simulink model "ata_xaui_2048pt_w32pnk"  (Simulink 6.2)
settings: Solver=ode45  StartTime=0.0  StopTime=20000  RelTol=1e-3
undefined symbols (not defined in the file): iBOB, pfb_coeff_gen_calc
libraries: xbsIndex_r3 x326, casper_library x37, xps_library x31, fft_library x1
(part 1 of 3)
settings Model: LastModifiedBy=siemion
settings DebuggingCC: SolverPrmCheckMsg=warning

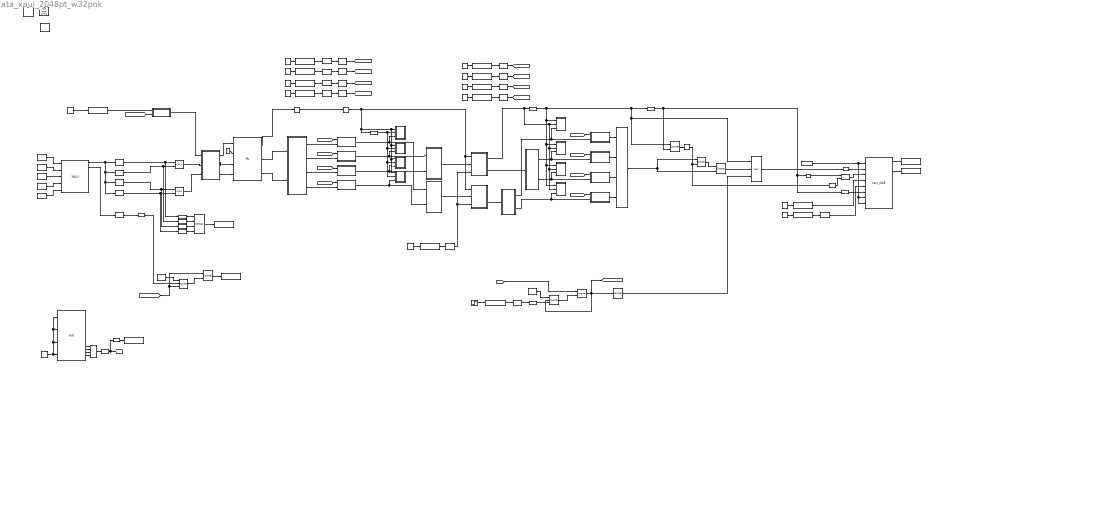
== system ata_xaui_2048pt_w32pnk ==
  note: left
  note: ATA Pulsar Machine
      | Author: Peter McMahon
      | Version: 1.0
      | February 2008
  note: n * LCM(taps*clksperFFT=2*2048=4096,
      | clksperacc=(acclen+1)*veclen=5*2048=10240)=20480
  note: XAUI Output:
      |
      | outofband[0]: 100PPS
      | outofband[1]: 1PPS
      |
      | data[0-7]: Pol 1 I
      | data[8-15]: Pol 1 Q
      | data[16-23]: Pol 2 I
      | data[24-31]: Pol 2 Q
      | data[31-63]: unused
  note: min acclen for serializer = # of parallel inputs
  note: XAUI Scope
      | Outputs raw bits from XAUI so you can measure voltage levels
  note: ARM/PPS Reset Circuit
      | 1. User sets ARM high at half-second
      | 2. 1PPS arrives.
      | 3. PPSARMReset signal goes high for one clock on the 1PPS
      | 4. ARM is reset, and won't go high again until user brings it low then high
  note: Unsigned, 18-bits, b.p. at 12
      | Coefficient by which to scale the output of the Stokes Detector.
  note: Extract 8 bits from 32
      | (latency: 1)
  note: When "valid" goes high, it's the start of a
      | packet, so insert a counter.
      |
      | Note that since the bitselect_i subsystems each have a delay of 1,
      | valid goes high 1 clock before the data arrives.
  note: Need valid to be high while data is valid (2048 clocks), and
      | one extra clock for the "header" (counter). Total clocks: 2049.
  note: Delay the valid and data signals so that
      | end-of-frame goes high for the last clock
      | that valid is high. This is a requirement for
      | the 10GbE block to work.
  note: ** Sending out data every second clock.
      | 10GbE tx_data input is 64 bits wide.
      | We only produce 32-bits of data per clock.
      | Therefore we must buffer 32-bits every second clock
      | and concat it with the current data output to get 64-bits
      | every second clock. The tx_valid line is modified to
      | accommodate this.
  note: Intended usage:
      | Connect to 108MHz bandwidth beamformer.
      | Input: I,Q 108MSa/sec, dual polarization.
      |   i.e. 8-bits I, 8-bits Q, x2 pol = 32 bits
      | Runs synchronously (i.e. assumes 32-bits
      | arrives from XAUI every FPGA clock)
  note: Selects which 8-bits from 32 are outputted.
      | 0 is lowest 8-bits.
      | 3 is highest 8-bits.
  note: Powers are unsigned and cross-terms are signed.
      | Hence we have to use separate accumulators for
      | them.
  note: The ADC serves two purposes:
      | 1.) Provide an external clock input so that the FPGA can be clocked at 108MHz.
      | 2.) Provide an input for 1PPS.
  note: 1PPS Delay
      |
      | Measures the delay between the 1PPS from the ADC and the
      | 1PPS from the XAUI (beamformer). This difference represents
      | the delay of the beamformer (in clock cycles of this design).
      |
      | The difference is only measured from the ARM/1PPS(ADC) - i.e. the
      | ARM register allows the ADC 1PPS to start the counter, and the counter
      | keeps track of how many clock pulses occur between this event and the
      | 1PPS emerging from the XAUI.
  note: PPSARMReset goes high when ARM has been set
      | and the 1PPS from the ADC goes high.
  note: Featuring:
      | 1. Saturation logic in the user "scale" blocks
      | 2. Output scopes
      | 3. 4-tap PFB
  " System Generator" : xbsIndex_r3/ System Generator  Tag=genX  xilinxfamily=Virtex2P  part=xc2vp50  speed=-7  package=ff1152  synthesis_tool=XST  directory=./ata_xaui_2048pt_with32bits/sysgen  testbench=off  simulink_period=1  sysclk_period=8  incr_netlist=off  trim_vbits=Everywhere in SubSystem  dbl_ovrd=According to Block Masks  core_generation=According to Block Masks  run_coregen=off  deprecated_control=off  eval_field=0
      settings: AttributesFormatString=System\nGenerator
  Constant : Constant  Value=4000
  Constant1 : Constant  Value=4000
  Constant2 : Constant  Value=2
  Constant{3..6} (4 alike) : Constant  Value=2^12
  Constant7 : Constant
  Constant8 : Constant
  Constant9 : Constant
  Slice : xbsIndex_r3/Slice  mode=Lower Bit Location + Width  nbits=20  bit1=0  base1=MSB of Input  bit0=0  base0=LSB of Input  boolean_output=off  explicit_period=off  period=1  dbl_ovrd=off
  Slice1 : xbsIndex_r3/Slice  mode=Lower Bit Location + Width  nbits=16  bit1=0  base1=MSB of Input  bit0=0  base0=LSB of Input  boolean_output=off  explicit_period=off  period=1  dbl_ovrd=off
  Slice{2,5..6,9} (4 alike) : xbsIndex_r3/Slice  mode=Lower Bit Location + Width  nbits=2  bit1=0  base1=MSB of Input  bit0=0  base0=LSB of Input  boolean_output=off  explicit_period=off  period=1  dbl_ovrd=off
  Slice{3..4,7..8} (4 alike) : xbsIndex_r3/Slice  mode=Lower Bit Location + Width  nbits=18  bit1=0  base1=MSB of Input  bit0=0  base0=LSB of Input  boolean_output=off  explicit_period=off  period=1  dbl_ovrd=off
  StokesDetector : Subsystem
  XAUI : xps_library/XAUI  Tag=xps:xaui  demux=1  port=iBOB:1  show_param=on  pre_emph=2  swing=800
  XSG core config : xps_library/XSG core config  Tag=xps:xsg  hw_sys=iBOB  ibob_linux=off  clk_src=adc0_clk  gpio_clk_io_group=iBOB:sma  gpio_clk_bit_index=0  clk_rate=125  sample_period=1  synthesis_tool=XST  mpc_type=powerpc405
  adc : xps_library/adc  Tag=xps:adc  adc_brd=iBOB:adc0  adc_clk_rate=500  adc_interleave=off  sample_period=1
  and_valid : xbsIndex_r3/Logical  logical_function=AND  inputs=2  precision=Full  arith_type=Unsigned  n_bits=8  bin_pt=2  align_bp=on  latency=0  explicit_period=off  period=1  en=off  dbl_ovrd=off  show_param=off
      settings: xl_area=[0, 0, 0, 0, 0, 0, 0]
  cns_10GbE : xbsIndex_r3/Constant  const=0  equ=P=C  arith_type=Boolean  n_bits=32  bin_pt=0  opselect=C  inp2=PCIN>>17  opr=+  inp1=P  carry=CIN  iostate=0  explicit_period=on  period=1  dbl_ovrd=off
  cns_1pps_delay : xbsIndex_r3/Constant  const=1  equ=P=C  arith_type=Boolean  n_bits=1  bin_pt=0  opselect=C  inp2=PCIN>>17  opr=+  inp1=P  carry=CIN  iostate=0  explicit_period=on  period=1  dbl_ovrd=off
  cns_acclen : Constant  Value=4
  cns_reset : xbsIndex_r3/Constant  const=1  equ=P=C  arith_type=Boolean  n_bits=1  bin_pt=0  opselect=C  inp2=PCIN>>17  opr=+  inp1=P  carry=CIN  iostate=0  explicit_period=on  period=1  dbl_ovrd=off
  cns_sync_period : Constant  Value=20480
  cns_xaui_rx_get : xbsIndex_r3/Constant  const=1  equ=P=C  arith_type=Boolean  n_bits=1  bin_pt=0  opselect=C  inp2=PCIN>>17  opr=+  inp1=P  carry=CIN  iostate=0  explicit_period=on  period=1  dbl_ovrd=off
  cns_xaui_rx_reset : xbsIndex_r3/Constant  const=0  equ=P=C  arith_type=Boolean  n_bits=1  bin_pt=0  opselect=C  inp2=PCIN>>17  opr=+  inp1=P  carry=CIN  iostate=0  explicit_period=on  period=1  dbl_ovrd=off
  cns_xaui_tx_data : xbsIndex_r3/Constant  const=0  equ=P=C  arith_type=Unsigned  n_bits=64  bin_pt=0  opselect=C  inp2=PCIN>>17  opr=+  inp1=P  carry=CIN  iostate=0  explicit_period=on  period=1  dbl_ovrd=off
  cns_xaui_tx_outofband : xbsIndex_r3/Constant  const=0  equ=P=C  arith_type=Unsigned  n_bits=8  bin_pt=0  opselect=C  inp2=PCIN>>17  opr=+  inp1=P  carry=CIN  iostate=0  explicit_period=on  period=1  dbl_ovrd=off
  cns_xaui_tx_valid : xbsIndex_r3/Constant  const=0  equ=P=C  arith_type=Boolean  n_bits=8  bin_pt=0  opselect=C  inp2=PCIN>>17  opr=+  inp1=P  carry=CIN  iostate=0  explicit_period=on  period=1  dbl_ovrd=off
  cnt_1pps_delay : xbsIndex_r3/Counter  cnt_type=Free Running  n_bits=32  bin_pt=0  arith_type=Unsigned  start_count=0  cnt_to=Inf  cnt_by_val=1  operation=Up  explicit_period=off  period=1  load_pin=off  rst=on  en=on  dbl_ovrd=off  show_param=off  use_rpm=on  gen_core=off
      settings: xl_area=[0, 0, 0, 0, 0, 0, 0]
  cnt_buffer : xbsIndex_r3/Counter  cnt_type=Free Running  n_bits=1  bin_pt=0  arith_type=Unsigned  start_count=1  cnt_to=Inf  cnt_by_val=1  operation=Up  explicit_period=off  period=1  load_pin=off  rst=on  en=on  dbl_ovrd=off  show_param=off  use_rpm=on  gen_core=off
      settings: xl_area=[0, 0, 0, 0, 0, 0, 0]
  coeff_delay : xbsIndex_r3/Delay  latency=6  reg_retiming=off  explicit_period=off  period=1  en=off  accept_only_valid=off  init_zero=on  dbl_ovrd=off  show_param=off
      settings: xl_area=[0, 0, 0, 0, 0, 0, 0]
  concat_buffer : xbsIndex_r3/Concat  num_inputs=2  explicit_period=off  period=1  dbl_ovrd=off
  concat_xauiscope : xbsIndex_r3/Concat  num_inputs=4  explicit_period=off  period=1  dbl_ovrd=off
  cram : Subsystem  AncestorBlock=gavrt_library/cram  mask(cram){num_slice=2}
      mask prompts: num_slice "Number of slices"
      mask help: Concatenates inputs together after forcing binary point to zero.
      mask init:
      | cram_init(gcb, ...
      |     'num_slice', num_slice);
  cram1 : Subsystem  AncestorBlock=gavrt_library/cram  mask(cram){num_slice=4}
      mask prompts: num_slice "Number of slices"
      mask help: Concatenates inputs together after forcing binary point to zero.
      mask init:
      | cram_init(gcb, ...
      |     'num_slice', num_slice);
  cram2 : Subsystem  AncestorBlock=gavrt_library/cram  mask(cram){num_slice=2}
      mask prompts: num_slice "Number of slices"
      mask help: Concatenates inputs together after forcing binary point to zero.
      mask init:
      | cram_init(gcb, ...
      |     'num_slice', num_slice);
  dly_10GbE_data : xbsIndex_r3/Delay  latency=1  reg_retiming=off  explicit_period=off  period=1  en=off  accept_only_valid=off  init_zero=on  dbl_ovrd=off  show_param=off
      settings: xl_area=[0, 0, 0, 0, 0, 0, 0]
  dly_10GbE_valid : xbsIndex_r3/Delay  latency=1  reg_retiming=on  explicit_period=off  period=1  en=off  accept_only_valid=off  init_zero=on  dbl_ovrd=off  show_param=off
      settings: xl_area=[0, 0, 0, 0, 0, 0, 0]
  fft1 : fft_library/fft  FFTSize=11  BitWidth=18  n_inputs=0  quantization=Truncate  overflow=Wrap  add_latency=3  mult_latency=4  bram_latency=3
      link override fft_biplex0/biplex_cplx_unscrambler/reorder/sync_delay/Constant: equ=P=C
      link override fft_biplex0/biplex_cplx_unscrambler/reorder/sync_delay/Constant1: equ=P=C
      link override fft_biplex0/biplex_cplx_unscrambler/reorder/sync_delay/Constant2: equ=P=C
      link override fft_biplex0/biplex_cplx_unscrambler/reorder/sync_delay/Constant3: equ=P=C
      link override fft_biplex0/biplex_cplx_unscrambler/reorder1/sync_delay/Constant: equ=P=C
      link override fft_biplex0/biplex_cplx_unscrambler/reorder1/sync_delay/Constant1: equ=P=C
      link override fft_biplex0/biplex_cplx_unscrambler/reorder1/sync_delay/Constant2: equ=P=C
      link override fft_biplex0/biplex_cplx_unscrambler/reorder1/sync_delay/Constant3: equ=P=C
      link override fft_biplex1/biplex_cplx_unscrambler/reorder/sync_delay/Constant: equ=P=C
      link override fft_biplex1/biplex_cplx_unscrambler/reorder/sync_delay/Constant1: equ=P=C
      link override fft_biplex1/biplex_cplx_unscrambler/reorder/sync_delay/Constant2: equ=P=C
      link override fft_biplex1/biplex_cplx_unscrambler/reorder/sync_delay/Constant3: equ=P=C
      link override fft_biplex1/biplex_cplx_unscrambler/reorder1/sync_delay/Constant: equ=P=C
      link override fft_biplex1/biplex_cplx_unscrambler/reorder1/sync_delay/Constant1: equ=P=C
      link override fft_biplex1/biplex_cplx_unscrambler/reorder1/sync_delay/Constant2: equ=P=C
      link override fft_biplex1/biplex_cplx_unscrambler/reorder1/sync_delay/Constant3: equ=P=C
  force_adc_i{0..3} (4 alike) : xbsIndex_r3/Reinterpret  force_arith_type=on  arith_type=Unsigned  force_bin_pt=on  bin_pt=0  force_valid=on
  ibob_lwip : xps_library/ibob_lwip
  inv_valid : xbsIndex_r3/Inverter  latency=0  explicit_period=off  period=1  en=off  dbl_ovrd=off  show_param=off
      settings: xl_area=[0, 0, 0, 0, 0, 0, 0]
  led0_10gbe_up : xps_library/gpio  Tag=xps:gpio  io_group=iBOB:led  io_dir=out  arith_type=Boolean  bitwidth=1  bin_pt=0  bit_index=1  sample_period=1  use_single_ended=off  use_ddr=off  reg_iob=on  reg_clk_phase=0  termination=None
  led1_10gbe_tx : xps_library/gpio  Tag=xps:gpio  io_group=iBOB:led  io_dir=out  arith_type=Boolean  bitwidth=1  bin_pt=0  bit_index=2  sample_period=1  use_single_ended=off  use_ddr=off  reg_iob=on  reg_clk_phase=0  termination=None
  led2_pps : xps_library/gpio  Tag=xps:gpio  io_group=iBOB:led  io_dir=out  arith_type=Boolean  bitwidth=1  bin_pt=0  bit_index=3  sample_period=1  use_single_ended=off  use_ddr=off  reg_iob=on  reg_clk_phase=0  termination=None
  log_arm_pps : xbsIndex_r3/Logical  logical_function=AND  inputs=2  precision=Full  arith_type=Unsigned  n_bits=8  bin_pt=2  align_bp=on  latency=0  explicit_period=off  period=1  en=off  dbl_ovrd=off  show_param=off
      settings: xl_area=[0, 0, 0, 0, 0, 0, 0]
  mux_counter_data : xbsIndex_r3/Mux  inputs=2  precision=Full  arith_type="Signed  (2's comp)"  n_bits=8  bin_pt=2  quantization=Truncate  overflow=Wrap  latency=1  explicit_period=off  period=1  en=off  dbl_ovrd=off  show_param=off  mux_type=off  use_rpm=off  gen_core=off
      settings: xl_area=[0, 0, 0, 0, 0, 0, 0]
  negedge1 : casper_library/Misc/negedge  Tag=Rising Edge Detector
  pfb_fir1 : Subsystem  AncestorBlock=casper_library/PFBs/pfb_fir  mask(pfb_fir){PFBSize=11, TotalTaps=4, WindowType=hamming, n_inputs=0, MakeBiplex=1, BitWidthIn=8, BitWidthOut=18, CoeffBitWidth=8, CoeffDistMem=1, add_latency=2, mult_latency=3, bram_latency=3, quantization=Truncate, fwidth=1}
      mask prompts: PFBSize "Size of PFB: (2^? pnts)"; TotalTaps "Total Number of Taps:"; WindowType "Windowing Function:"; n_inputs "Number of Simultaneous Inputs: (2^?)"; MakeBiplex "Make Biplex"; BitWidthIn "Input Bitwidth:"; BitWidthOut "Output Bitwidth:"; CoeffBitWidth "Coefficient Bitwidth:"; CoeffDistMem "Use Distributed Memory for Coeffs"; add_latency "Add Latency"; mult_latency "Mult Latency"; bram_latency "BRAM Latency"; quantization "Quantization Behavior"; fwidth "Bin Width Scaling (normal=1)"
      mask init:
      | pfb_fir_init(gcb, ...
      |     'PFBSize', PFBSize, ...
      |     'TotalTaps', TotalTaps, ...
      |     'WindowType', WindowType, ...
      |     'n_inputs', n_inputs, ...
      |     'MakeBiplex', MakeBiplex, ...
      |     'BitWidthIn', BitWidthIn, ...
      |     'BitWidthOut', BitWidthOut, ...
      |     'CoeffBitWidth', CoeffBitWidth, ...
      |     'CoeffDistMem', CoeffDistMem, ...
      |     'add_latency', add_latency, ...
      |     'mult_latency', mult_latency, ...
      |     'bram_latency', bram_latency, ...
      |     'quantization', quantization, ...
      |     'fwidth', fwidth);
      settings: AttributesFormatString=taps=4, add_latency=2
      mask StyleString: edit,edit,popup(bartlett|barthannwin|blackman|blackmanharris|bohamwin|chebwin|flattopwin|gausswin|hamming|hann|kaiser|nuttallwin|parzenwin|rectwin|tukeywin|triang),edit,edit,edit,edit,edit,edit,edit,edit,edit,popup(Truncate|Round  (unbiased: +/- Inf)|Round  (unbiased: Even Values)),edit
  posedge : casper_library/Misc/posedge  Tag=Rising Edge Detector
  posedge_arm : casper_library/Misc/posedge  Tag=Rising Edge Detector
  posedge_pps : casper_library/Misc/posedge  Tag=Rising Edge Detector
  posedge_pps_xaui : casper_library/Misc/posedge  Tag=Rising Edge Detector
  pulse_ext : casper_library/Misc/pulse_ext  pulse_len=2049
  pulse_ext1 : casper_library/Misc/pulse_ext  pulse_len=2^22
  pulse_ext2 : casper_library/Misc/pulse_ext  pulse_len=2048
  reg_10GbE_destport0 : xps_library/software register  Tag=xps:sw_reg  io_dir=From Processor  arith_type=Unsigned  bitwidth=32  bin_pt=0  sample_period=1  gw_name=ata_xaui_2048pt_w32pnk_reg_10GbE_destport0_user_data_out
  reg_1pps_delay : xbsIndex_r3/Register  init=0  reg_only_valid=off  explicit_period=off  period=1  rst=on  en=on  out_en=off  dbl_ovrd=off  show_param=off
      settings: xl_area=[0, 0, 0, 0, 0, 0, 0]
  reg_1ppsdelay : xps_library/software register  Tag=xps:sw_reg  io_dir=To Processor  arith_type=Unsigned  bitwidth=32  bin_pt=0  sample_period=1  gw_name=ata_xaui_2048pt_w32pnk_reg_1ppsdelay_user_data_in
  reg_acclen : xps_library/software register  Tag=xps:sw_reg  io_dir=From Processor  arith_type=Unsigned  bitwidth=32  bin_pt=0  sample_period=1  gw_name=ata_xaui_2048pt_w32pnk_reg_acclen_user_data_out
  reg_arm : xps_library/software register  Tag=xps:sw_reg  io_dir=From Processor  arith_type=Unsigned  bitwidth=32  bin_pt=0  sample_period=1  gw_name=ata_xaui_2048pt_w32pnk_reg_arm_user_data_out
  reg_buffer : xbsIndex_r3/Register  init=0  reg_only_valid=off  explicit_period=off  period=1  rst=off  en=on  out_en=off  dbl_ovrd=off  show_param=off
      settings: xl_area=[0, 0, 0, 0, 0, 0, 0]
  reg_coeff_stokes1 : xps_library/software register  Tag=xps:sw_reg  io_dir=From Processor  arith_type=Unsigned  bitwidth=32  bin_pt=0  sample_period=1  gw_name=ata_xaui_2048pt_w32pnk_reg_coeff_stokes1_user_data_out
  reg_coeff_stokes2 : xps_library/software register  Tag=xps:sw_reg  io_dir=From Processor  arith_type=Unsigned  bitwidth=32  bin_pt=0  sample_period=1  gw_name=ata_xaui_2048pt_w32pnk_reg_coeff_stokes2_user_data_out
  reg_coeff_stokes3 : xps_library/software register  Tag=xps:sw_reg  io_dir=From Processor  arith_type=Unsigned  bitwidth=32  bin_pt=0  sample_period=1  gw_name=ata_xaui_2048pt_w32pnk_reg_coeff_stokes3_user_data_out
  reg_coeff_stokes4 : xps_library/software register  Tag=xps:sw_reg  io_dir=From Processor  arith_type=Unsigned  bitwidth=32  bin_pt=0  sample_period=1  gw_name=ata_xaui_2048pt_w32pnk_reg_coeff_stokes4_user_data_out
  reg_ip : xps_library/software register  Tag=xps:sw_reg  io_dir=From Processor  arith_type=Unsigned  bitwidth=32  bin_pt=0  sample_period=1  gw_name=ata_xaui_2048pt_w32pnk_reg_ip_user_data_out
  reg_output_bitselect1 : xps_library/software register  Tag=xps:sw_reg  io_dir=From Processor  arith_type=Unsigned  bitwidth=32  bin_pt=0  sample_period=1  gw_name=ata_xaui_2048pt_w32pnk_reg_output_bitselect1_user_data_out
  reg_output_bitselect2 : xps_library/software register  Tag=xps:sw_reg  io_dir=From Processor  arith_type=Unsigned  bitwidth=32  bin_pt=0  sample_period=1  gw_name=ata_xaui_2048pt_w32pnk_reg_output_bitselect2_user_data_out
  reg_output_bitselect3 : xps_library/software register  Tag=xps:sw_reg  io_dir=From Processor  arith_type=Unsigned  bitwidth=32  bin_pt=0  sample_period=1  gw_name=ata_xaui_2048pt_w32pnk_reg_output_bitselect3_user_data_out
  reg_output_bitselect4 : xps_library/software register  Tag=xps:sw_reg  io_dir=From Processor  arith_type=Unsigned  bitwidth=32  bin_pt=0  sample_period=1  gw_name=ata_xaui_2048pt_w32pnk_reg_output_bitselect4_user_data_out
  reg_reset_arm : xbsIndex_r3/Register  init=0  reg_only_valid=off  explicit_period=on  period=1  rst=on  en=on  out_en=off  dbl_ovrd=off  show_param=off
      settings: xl_area=[0, 0, 0, 0, 0, 0, 0]
  reg_sync_period : xps_library/software register  Tag=xps:sw_reg  io_dir=From Processor  arith_type=Unsigned  bitwidth=32  bin_pt=0  sample_period=1  gw_name=ata_xaui_2048pt_w32pnk_reg_sync_period_user_data_out
  reg_xauiscope : xps_library/software register  Tag=xps:sw_reg  io_dir=To Processor  arith_type=Unsigned  bitwidth=32  bin_pt=0  sample_period=1  gw_name=ata_xaui_2048pt_w32pnk_reg_xauiscope_user_data_in
  reint{,1..3} (4 alike) : xbsIndex_r3/Reinterpret  force_arith_type=on  arith_type=Unsigned  force_bin_pt=on  bin_pt=12  force_valid=on
  ri_to_c1 : casper_library/Misc/ri_to_c
  ri_to_c2 : casper_library/Misc/ri_to_c
  scope_s_output2 : Subsystem
  scope_s_output3 : Subsystem
  scope_s_scaled1 : Subsystem
  scope_s_scaled2 : Subsystem
  scope_u_output1 : Subsystem
  scope_u_output4 : Subsystem
  scope_u_scaled1 : Subsystem
  scope_u_scaled2 : Subsystem
  shift : xbsIndex_r3/Constant  const=-1  equ=P=C  arith_type="Signed  (2's comp)"  n_bits=32  bin_pt=0  opselect=C  inp2=PCIN>>17  opr=+  inp1=P  carry=CIN  iostate=0  explicit_period=on  period=1  dbl_ovrd=off
  signed_bitselect_2 : Subsystem
  signed_bitselect_3 : Subsystem
  signed_scale2 : Subsystem
  signed_scale3 : Subsystem
  sim_step_arm : Step  SampleTime=0
  sim_zero : Constant  Value=0
  slc_arm : xbsIndex_r3/Slice  mode=Lower Bit Location + Width  nbits=1  bit1=0  base1=MSB of Input  bit0=0  base0=LSB of Input  boolean_output=on  explicit_period=off  period=1  dbl_ovrd=off
  slc_xaui_data_pol1_I : xbsIndex_r3/Slice  mode=Lower Bit Location + Width  nbits=8  bit1=0  base1=MSB of Input  bit0=0  base0=LSB of Input  boolean_output=off  explicit_period=off  period=1  dbl_ovrd=off
  slc_xaui_data_pol1_Q : xbsIndex_r3/Slice  mode=Lower Bit Location + Width  nbits=8  bit1=0  base1=MSB of Input  bit0=8  base0=LSB of Input  boolean_output=off  explicit_period=off  period=1  dbl_ovrd=off
  slc_xaui_data_pol2_I : xbsIndex_r3/Slice  mode=Lower Bit Location + Width  nbits=8  bit1=0  base1=MSB of Input  bit0=16  base0=LSB of Input  boolean_output=off  explicit_period=off  period=1  dbl_ovrd=off
  slc_xaui_data_pol2_Q : xbsIndex_r3/Slice  mode=Lower Bit Location + Width  nbits=8  bit1=0  base1=MSB of Input  bit0=24  base0=LSB of Input  boolean_output=off  explicit_period=off  period=1  dbl_ovrd=off
  slc_xaui_outofband_1pps : xbsIndex_r3/Slice  mode=Lower Bit Location + Width  nbits=1  bit1=0  base1=MSB of Input  bit0=1  base0=LSB of Input  boolean_output=on  explicit_period=off  period=1  dbl_ovrd=off
  slice_buffer : xbsIndex_r3/Slice  mode=Lower Bit Location + Width  nbits=1  bit1=0  base1=MSB of Input  bit0=0  base0=LSB of Input  boolean_output=on  explicit_period=off  period=1  dbl_ovrd=off
  stokes_delay : xbsIndex_r3/Delay  latency=5  reg_retiming=off  explicit_period=off  period=1  en=off  accept_only_valid=off  init_zero=on  dbl_ovrd=off  show_param=off
      settings: xl_area=[0, 0, 0, 0, 0, 0, 0]
  sync_generator : Subsystem
  sync_or : xbsIndex_r3/Logical  logical_function=OR  inputs=4  precision=Full  arith_type=Unsigned  n_bits=8  bin_pt=2  align_bp=on  latency=1  explicit_period=off  period=1  en=off  dbl_ovrd=off  show_param=off
      settings: xl_area=[0, 0, 0, 0, 0, 0, 0]
  system_counter : xbsIndex_r3/Counter  cnt_type=Free Running  n_bits=64  bin_pt=0  arith_type=Unsigned  start_count=0  cnt_to=Inf  cnt_by_val=1  operation=Up  explicit_period=off  period=1  load_pin=off  rst=on  en=off  dbl_ovrd=off  show_param=off  use_rpm=on  gen_core=off
      settings: xl_area=[0, 0, 0, 0, 0, 0, 0]
  ten_GbE0 : xps_library/ten_GbE  Tag=xps:tengbe  port=iBOB:0  mac_lite=off  show_param=on  pre_emph=2  swing=800
  uncram_crossterms : Subsystem  AncestorBlock=gavrt_library/uncram  mask(uncram){num_slice=2, slice_width=32, bin_pt=23, arith_type=1}
      mask prompts: num_slice "Number of slices"; slice_width "Slice Width"; bin_pt "Output Binary Point"; arith_type "Output Arithmetic Type (0=Unsigned, 1=Signed, 2=Boolean)"
      mask help: Takes a concatenated input and slices it up into even pieces and reinterprets them as signed fixed point numbers with a given binary point.
      mask init:
      | uncram_init(gcb, ...
      |     'num_slice', num_slice, ...
      |     'slice_width', slice_width, ...
      |     'bin_pt', bin_pt, ...
      |     'arith_type', arith_type);
      settings: AttributesFormatString=Fix_32_23
  uncram_powers : Subsystem  AncestorBlock=gavrt_library/uncram  mask(uncram){num_slice=2, slice_width=32, bin_pt=23, arith_type=0}
      mask prompts: num_slice "Number of slices"; slice_width "Slice Width"; bin_pt "Output Binary Point"; arith_type "Output Arithmetic Type (0=Unsigned, 1=Signed, 2=Boolean)"
      mask help: Takes a concatenated input and slices it up into even pieces and reinterprets them as signed fixed point numbers with a given binary point.
      mask init:
      | uncram_init(gcb, ...
      |     'num_slice', num_slice, ...
      |     'slice_width', slice_width, ...
      |     'bin_pt', bin_pt, ...
      |     'arith_type', arith_type);
      settings: AttributesFormatString=UFix_32_23
  unsigned_bitselect_1 : Subsystem
  unsigned_bitselect_4 : Subsystem
  unsigned_scale1 : Subsystem
  unsigned_scale2 : Subsystem
  vacc : Subsystem  AncestorBlock=gavrt_library/vacc  mask(vacc){veclen=11, ninputs=2, max_accum=8, arith_type=1, in_bit_width=24, in_bin_pt=23, out_bit_width=32, out_bin_pt=23, register_din=1, add_latency=2, bram_latency=2, mux_latency=1}
      mask prompts: veclen "Vector Length (2^?)"; ninputs "Number of Simultaneous Vectors"; max_accum "Maximum # Accumulations (2^?)"; arith_type "Arithmetic Type (0=Unsigned, 1=Signed)"; in_bit_width "Input Bit Width"; in_bin_pt "Input Binary Point"; out_bit_width "Output Bit Width"; out_bin_pt "Output Binary Point"; register_din "Register Input Data  (1 = Enable Register Retiming on input delay)"; add_latency "Add Latency"; bram_latency "BRAM Latency"; mux_latency "Mux Latency"
      mask help:
      | Sync is expected the clock before the first data to be accumulated.
      | Use the Cram block to feed din for multiple simultaneous inputs.
      | acc_len is the number of vectors to sum.
      | valid is high while a valid accumulation is being clocked out on dout.
      | If only one sync pulse is provided, valid accumulations will repeatedly appear on dout as they become available.
      | Undesired behavior may occur if acc_len is changed without a new sync pulse.
      | Note: The output is an unsigned concatenation of the output streams. Thus, even with only one stream, the output must be recast before using.
      | Register Input Data controls the "Enable Register Retiming" parameter of the delays on 'din'.
      mask init:
      | vacc_init(gcb, ...
      |     'veclen', veclen, ...
      |     'ninputs', ninputs, ...
      |     'max_accum', max_accum, ...
      |     'arith_type', arith_type, ...
      |     'in_bit_width', in_bit_width, ...
      |     'in_bin_pt', in_bin_pt, ...
      |     'out_bit_width', out_bit_width, ...
      |     'out_bin_pt', out_bin_pt, ...
      |     'register_din', register_din, ...
      |     'add_latency', add_latency, ...
      |     'bram_latency', bram_latency, ...
      |     'mux_latency', mux_latency);
      settings: AttributesFormatString=|
      | vector length=2048, inputs=2
      | max accumulations=2^8
  vacc1 : Subsystem  AncestorBlock=gavrt_library/vacc  mask(vacc){veclen=11, ninputs=2, max_accum=8, arith_type=0, in_bit_width=24, in_bin_pt=23, out_bit_width=32, out_bin_pt=23, register_din=1, add_latency=2, bram_latency=2, mux_latency=1}
      mask prompts: veclen "Vector Length (2^?)"; ninputs "Number of Simultaneous Vectors"; max_accum "Maximum # Accumulations (2^?)"; arith_type "Arithmetic Type (0=Unsigned, 1=Signed)"; in_bit_width "Input Bit Width"; in_bin_pt "Input Binary Point"; out_bit_width "Output Bit Width"; out_bin_pt "Output Binary Point"; register_din "Register Input Data  (1 = Enable Register Retiming on input delay)"; add_latency "Add Latency"; bram_latency "BRAM Latency"; mux_latency "Mux Latency"
      mask help:
      | Sync is expected the clock before the first data to be accumulated.
      | Use the Cram block to feed din for multiple simultaneous inputs.
      | acc_len is the number of vectors to sum.
      | valid is high while a valid accumulation is being clocked out on dout.
      | If only one sync pulse is provided, valid accumulations will repeatedly appear on dout as they become available.
      | Undesired behavior may occur if acc_len is changed without a new sync pulse.
      | Note: The output is an unsigned concatenation of the output streams. Thus, even with only one stream, the output must be recast before using.
      | Register Input Data controls the "Enable Register Retiming" parameter of the delays on 'din'.
      mask init: same as ata_xaui_2048pt_w32pnk/vacc
      settings: AttributesFormatString=|
      | vector length=2048, inputs=2
      | max accumulations=2^8
  wires:
  Slice/1 -> vacc/3(acc_len), vacc1/3(acc_len)
  stokes_delay/1 -> coeff_delay/1
  reg_sync_period/1 -> sync_generator/1(period)
  sim_zero/1 -> adc/4, adc/3, adc/2, adc/1
  sync_generator/1(sync) -> pfb_fir1/1(sync)
  reg_acclen/1 -> Slice/1
  cns_acclen/1 -> reg_acclen/1
  cns_sync_period/1 -> reg_sync_period/1
  adc/13 -> sync_or/1
  adc/14 -> sync_or/2
  adc/15 -> sync_or/3
  adc/16 -> sync_or/4
  sync_or/1 -> posedge_pps/1
  ten_GbE0/1 -> led0_10gbe_up/1
  reg_10GbE_destport0/1 -> Slice1/1
  Constant/1 -> reg_10GbE_destport0/1
  Slice1/1 -> ten_GbE0/5
  Constant1/1 -> reg_ip/1
  reg_ip/1 -> ten_GbE0/4
  cns_10GbE/1 -> ten_GbE0/1, ten_GbE0/8, ten_GbE0/7
  posedge_pps/1 -> [PPS], pulse_ext1/1
  [PPSARMReset] -> sync_generator/2(reset)
  ten_GbE0/3 -> led1_10gbe_tx/1
  pulse_ext1/1 -> led2_pps/1
  reg_arm/1 -> slc_arm/1
  cns_reset/1 -> reg_reset_arm/1
  reg_reset_arm/1 -> log_arm_pps/2
  [PPS] -> log_arm_pps/1
  log_arm_pps/1 -> reg_reset_arm/2, system_counter/1, [PPSARMReset]
  slc_arm/1 -> posedge_arm/1
  posedge_arm/1 -> reg_reset_arm/3
  concat_xauiscope/1 -> reg_xauiscope/1
  force_adc_i0/1 -> concat_xauiscope/1
  force_adc_i1/1 -> concat_xauiscope/2
  force_adc_i2/1 -> concat_xauiscope/3
  force_adc_i3/1 -> concat_xauiscope/4
  sim_step_arm/1 -> reg_arm/1
  Constant3/1 -> reg_coeff_stokes1/1
  reg_coeff_stokes1/1 -> Slice3/1
  Slice3/1 -> reint/1
  signed_bitselect_2/1(data_out) -> cram1/2(In2)
  signed_bitselect_3/1(data_out) -> cram1/3(In3)
  unsigned_bitselect_4/1(data_out) -> cram1/4(In4)
  vacc/1(valid) -> posedge/1, scope_u_output1/2(en), scope_s_output2/2(en), scope_s_output3/2(en), scope_u_output4/2(en)
  system_counter/1 -> mux_counter_data/3
  posedge/1 -> mux_counter_data/1, cnt_buffer/1, pulse_ext/1, scope_u_output1/1(rst), scope_s_output2/1(rst), scope_u_output4/1(rst), scope_s_output3/1(rst)
  pulse_ext/1 -> cnt_buffer/2, dly_10GbE_valid/1, negedge1/1
  negedge1/1 -> ten_GbE0/6
  dly_10GbE_data/1 -> ten_GbE0/2
  reg_buffer/1 -> concat_buffer/1
  cnt_buffer/1 -> slice_buffer/1
  slice_buffer/1 -> reg_buffer/2, inv_valid/1
  mux_counter_data/1 -> dly_10GbE_data/1
  concat_buffer/1 -> mux_counter_data/2
  cram1/1(Out) -> concat_buffer/2, reg_buffer/1
  inv_valid/1 -> and_valid/2
  dly_10GbE_valid/1 -> and_valid/1
  and_valid/1 -> ten_GbE0/3
  ri_to_c2/1 -> pfb_fir1/2(pol1_in1)
  ri_to_c1/1 -> pfb_fir1/3(pol2_in1)
  pfb_fir1/1(sync_out) -> fft1/1
  shift/1 -> fft1/2
  pfb_fir1/2(pol1_out1) -> fft1/3
  pfb_fir1/3(pol2_out1) -> fft1/4
  fft1/1 -> stokes_delay/1
  fft1/2 -> StokesDetector/1(pol1_f0)
  fft1/3 -> StokesDetector/2(pol2_f0)
  coeff_delay/1 -> vacc/1(sync), vacc1/1(sync), scope_u_scaled1/1(rst), scope_u_scaled2/1(rst), scope_s_scaled1/1(rst), scope_s_scaled2/1(rst), pulse_ext2/1
  StokesDetector/1(f0_pol1_pow) -> unsigned_scale1/2(data_in)
  StokesDetector/2(f0_x_re) -> signed_scale2/2(data_in)
  StokesDetector/3(f0_x_im) -> signed_scale3/2(data_in)
  StokesDetector/4(f0_pol2_pow) -> unsigned_scale2/2(data_in)
  reint/1 -> [StokesCoeff1]
  Constant4/1 -> reg_coeff_stokes2/1
  reg_coeff_stokes2/1 -> Slice4/1
  Slice4/1 -> reint1/1
  reint1/1 -> [StokesCoeff2]
  Constant5/1 -> reg_coeff_stokes3/1
  reg_coeff_stokes3/1 -> Slice7/1
  Slice7/1 -> reint2/1
  reint2/1 -> [StokesCoeff3]
  Constant6/1 -> reg_coeff_stokes4/1
  reg_coeff_stokes4/1 -> Slice8/1
  Slice8/1 -> reint3/1
  reint3/1 -> [StokesCoeff4]
  [StokesCoeff1] -> unsigned_scale1/1(coeff)
  [StokesCoeff2] -> signed_scale2/1(coeff)
  [StokesCoeff3] -> signed_scale3/1(coeff)
  [StokesCoeff4] -> unsigned_scale2/1(coeff)
  Constant2/1 -> reg_output_bitselect1/1
  reg_output_bitselect1/1 -> Slice2/1
  signed_scale2/1(data_out) -> scope_s_scaled2/3(data_in), cram2/1(In1)
  signed_scale3/1(data_out) -> scope_s_scaled1/3(data_in), cram2/2(In2)
  cram2/1(Out) -> vacc/2(din)
  cram/1(Out) -> vacc1/2(din)
  unsigned_scale1/1(data_out) -> scope_u_scaled1/3(data_in), cram/1(In1)
  unsigned_scale2/1(data_out) -> scope_u_scaled2/3(data_in), cram/2(In2)
  uncram_crossterms/1(Out1) -> signed_bitselect_2/2(data_in), scope_s_output2/3(data_in)
  uncram_crossterms/2(Out2) -> signed_bitselect_3/2(data_in), scope_s_output3/3(data_in)
  vacc/2(dout) -> uncram_crossterms/1(In)
  vacc1/2(dout) -> uncram_powers/1(In)
  uncram_powers/1(Out1) -> unsigned_bitselect_1/2(data_in), scope_u_output1/3(data_in)
  unsigned_bitselect_1/1(data_out) -> cram1/1(In1)
  Constant7/1 -> reg_output_bitselect2/1
  reg_output_bitselect2/1 -> Slice5/1
  Constant8/1 -> reg_output_bitselect3/1
  reg_output_bitselect3/1 -> Slice6/1
  Constant9/1 -> reg_output_bitselect4/1
  reg_output_bitselect4/1 -> Slice9/1
  Slice2/1 -> [BitSelect1]
  Slice5/1 -> [BitSelect2]
  Slice6/1 -> [BitSelect3]
  Slice9/1 -> [BitSelect4]
  [BitSelect1] -> unsigned_bitselect_1/1(bitselect)
  uncram_powers/2(Out2) -> unsigned_bitselect_4/2(data_in), scope_u_output4/3(data_in)
  [BitSelect4] -> unsigned_bitselect_4/1(bitselect)
  [BitSelect3] -> signed_bitselect_3/1(bitselect)
  [BitSelect2] -> signed_bitselect_2/1(bitselect)
  XAUI/1 -> slc_xaui_data_pol1_I/1, slc_xaui_data_pol1_Q/1, slc_xaui_data_pol2_I/1, slc_xaui_data_pol2_Q/1
  slc_xaui_data_pol1_I/1 -> force_adc_i0/1, ri_to_c2/1
  slc_xaui_data_pol1_Q/1 -> force_adc_i1/1, ri_to_c2/2
  slc_xaui_data_pol2_I/1 -> force_adc_i2/1, ri_to_c1/1
  slc_xaui_data_pol2_Q/1 -> force_adc_i3/1, ri_to_c1/2
  cns_xaui_rx_get/1 -> XAUI/1
  cns_xaui_rx_reset/1 -> XAUI/2
  cns_xaui_tx_data/1 -> XAUI/3
  cns_xaui_tx_outofband/1 -> XAUI/4
  cns_xaui_tx_valid/1 -> XAUI/5
  slc_xaui_outofband_1pps/1 -> posedge_pps_xaui/1
  XAUI/2 -> slc_xaui_outofband_1pps/1
  cnt_1pps_delay/1 -> reg_1ppsdelay/1
  cns_1pps_delay/1 -> reg_1pps_delay/1
  [PPSARMReset] -> reg_1pps_delay/3, cnt_1pps_delay/1
  reg_1pps_delay/1 -> cnt_1pps_delay/2
  posedge_pps_xaui/1 -> reg_1pps_delay/2
  pulse_ext2/1 -> scope_u_scaled1/2(en), scope_s_scaled2/2(en), scope_s_scaled1/2(en), scope_u_scaled2/2(en)

== system ata_xaui_2048pt_w32pnk/StokesDetector ==
  pol1_f0 : Inport  Port=1  LatchInput=off
  pol2_f0 : Inport  Port=2  LatchInput=off
  XMultiply_f0 : Subsystem
  pol1_power0 : Subsystem
  pol2_power0 : Subsystem
  f0_pol1_pow : Outport
  f0_x_re : Outport  Port=2
  f0_x_im : Outport  Port=3
  f0_pol2_pow : Outport  Port=4
  wires:
  pol1_f0/1 -> XMultiply_f0/1(Pol1), pol1_power0/1(c)
  pol2_f0/1 -> XMultiply_f0/2(Pol2), pol2_power0/1(c)
  pol1_power0/1(power) -> f0_pol1_pow/1
  XMultiply_f0/1(X Real) -> f0_x_re/1
  XMultiply_f0/2(X Imag) -> f0_x_im/1
  pol2_power0/1(power) -> f0_pol2_pow/1

== system ata_xaui_2048pt_w32pnk/cram ==
  In1 : Inport  Port=1  LatchInput=off
  In2 : Inport  Port=2  LatchInput=off
  Concat : S-Function  AncestorBlock=xbsIndex_r3/Concat  FunctionName=xlconcat  Parameters=sfcn_mwsv__  mask(Xilinx Bus Concatenator){num_inputs=2, explicit_period=off, period=1, dbl_ovrd=off}
      mask prompts: num_inputs "Number of Inputs"; explicit_period "Use Explicit Sample Period"; period "Sample Period  (use -1 to inherit first known input period)"; dbl_ovrd "Override with Doubles"
      mask help: Concatenates two or more inputs. Inputs must be unsigned with binary point at zero.
      mask init:
      | [designRoot, family, part, speed, package, simulinkPeriod, sysclkPeriod, dbl_ovrd, trimVbit] = xlSysgenSettings(gcb,1,1);
      | [bg,fg] = xlcmap('XBlock',dbl_ovrd);
      | iPos = get_param(gcb,'Position');
      | iWidth=iPos(3)-iPos(1); iHeight=iPos(4)-iPos(2);
      | iCx=iWidth/2;
      | iCy=iHeight/2;
      | [logoX, logoY] = xlogo(iPos);
      | 
      | 
      | 
      | 
      | % one time added for param list
      | numInputs = num_inputs + 1;
      | precision0 = 1;
      | latency = 0;
      | dblOvrd = dbl_ovrd;
      | explicitClk = explicit_period;
      | 
      | 
      | % just pass everything to s-function
      | sfcn_mwsv__ = get_param(gcb, 'MaskWSVariables');
      mask Help: eval('xlWeb(xlhtmldoclink(''Concat''))');
      mask StyleString: popup(2|3|4|5|6|7|8|9|10|11|12|13|14|15|16),checkbox,edit,checkbox
      mask CallbackString: |xlMagicCallback||
      mask Display:
      | patch([0 iWidth iWidth 0],[0 0 iHeight iHeight] , bg);
      | patch(logoX,logoY, fg);
      | port_label('input',1,'hi');
      | port_label('input',num_inputs+1,'lo');
      | port_label('output',1,'cat');
      | ;plot([0 0 iWidth iWidth 0], [0 iHeight iHeight 0 0]);
  Reinterp1 : xbsIndex_r3/Reinterpret  force_arith_type=on  arith_type=Unsigned  force_bin_pt=on  bin_pt=0  force_valid=on
  Reinterp2 : xbsIndex_r3/Reinterpret  force_arith_type=on  arith_type=Unsigned  force_bin_pt=on  bin_pt=0  force_valid=on
  Out : Outport
  wires:
  Concat/1 -> Out/1
  In1/1 -> Reinterp1/1
  Reinterp1/1 -> Concat/1
  In2/1 -> Reinterp2/1
  Reinterp2/1 -> Concat/2

== system ata_xaui_2048pt_w32pnk/cram1 ==
  In1 : Inport  Port=1  LatchInput=off
  In2 : Inport  Port=2  LatchInput=off
  In3 : Inport  Port=3  LatchInput=off
  In4 : Inport  Port=4  LatchInput=off
  Concat : S-Function  AncestorBlock=xbsIndex_r3/Concat  FunctionName=xlconcat  Parameters=sfcn_mwsv__  mask(Xilinx Bus Concatenator){num_inputs=4, explicit_period=off, period=1, dbl_ovrd=off}
      mask prompts: num_inputs "Number of Inputs"; explicit_period "Use Explicit Sample Period"; period "Sample Period  (use -1 to inherit first known input period)"; dbl_ovrd "Override with Doubles"
      mask help: Concatenates two or more inputs. Inputs must be unsigned with binary point at zero.
      mask init: same as ata_xaui_2048pt_w32pnk/cram/Concat
      mask Help: eval('xlWeb(xlhtmldoclink(''Concat''))');
      mask StyleString: popup(2|3|4|5|6|7|8|9|10|11|12|13|14|15|16),checkbox,edit,checkbox
      mask CallbackString: |xlMagicCallback||
      mask Display:
      | patch([0 iWidth iWidth 0],[0 0 iHeight iHeight] , bg);
      | patch(logoX,logoY, fg);
      | port_label('input',1,'hi');
      | port_label('input',num_inputs+1,'lo');
      | port_label('output',1,'cat');
      | ;plot([0 0 iWidth iWidth 0], [0 iHeight iHeight 0 0]);
  Reinterp{1..4} (4 alike) : xbsIndex_r3/Reinterpret  force_arith_type=on  arith_type=Unsigned  force_bin_pt=on  bin_pt=0  force_valid=on
  Out : Outport
  wires:
  Concat/1 -> Out/1
  In1/1 -> Reinterp1/1
  Reinterp1/1 -> Concat/1
  In2/1 -> Reinterp2/1
  Reinterp2/1 -> Concat/2
  In3/1 -> Reinterp3/1
  Reinterp3/1 -> Concat/3
  In4/1 -> Reinterp4/1
  Reinterp4/1 -> Concat/4

== system ata_xaui_2048pt_w32pnk/cram2 ==
  In1 : Inport  Port=1  LatchInput=off
  In2 : Inport  Port=2  LatchInput=off
  Concat : S-Function  AncestorBlock=xbsIndex_r3/Concat  FunctionName=xlconcat  Parameters=sfcn_mwsv__  mask(Xilinx Bus Concatenator){num_inputs=2, explicit_period=off, period=1, dbl_ovrd=off}
      mask prompts: num_inputs "Number of Inputs"; explicit_period "Use Explicit Sample Period"; period "Sample Period  (use -1 to inherit first known input period)"; dbl_ovrd "Override with Doubles"
      mask help: Concatenates two or more inputs. Inputs must be unsigned with binary point at zero.
      mask init: same as ata_xaui_2048pt_w32pnk/cram/Concat
      mask Help: eval('xlWeb(xlhtmldoclink(''Concat''))');
      mask StyleString: popup(2|3|4|5|6|7|8|9|10|11|12|13|14|15|16),checkbox,edit,checkbox
      mask CallbackString: |xlMagicCallback||
      mask Display:
      | patch([0 iWidth iWidth 0],[0 0 iHeight iHeight] , bg);
      | patch(logoX,logoY, fg);
      | port_label('input',1,'hi');
      | port_label('input',num_inputs+1,'lo');
      | port_label('output',1,'cat');
      | ;plot([0 0 iWidth iWidth 0], [0 iHeight iHeight 0 0]);
  Reinterp1 : xbsIndex_r3/Reinterpret  force_arith_type=on  arith_type=Unsigned  force_bin_pt=on  bin_pt=0  force_valid=on
  Reinterp2 : xbsIndex_r3/Reinterpret  force_arith_type=on  arith_type=Unsigned  force_bin_pt=on  bin_pt=0  force_valid=on
  Out : Outport
  wires:
  Reinterp2/1 -> Concat/2
  In2/1 -> Reinterp2/1
  Reinterp1/1 -> Concat/1
  In1/1 -> Reinterp1/1
  Concat/1 -> Out/1

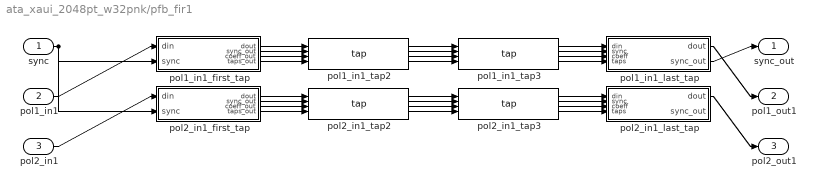
== system ata_xaui_2048pt_w32pnk/pfb_fir1 ==
  sync : Inport  Port=1  LatchInput=off
  pol1_in1 : Inport  Port=2  LatchInput=off
  pol2_in1 : Inport  Port=3  LatchInput=off
  pol1_in1_first_tap : Subsystem  AncestorBlock=casper_library/PFBs/first_tap  mask(first_tap){nput=0, PFBSize=11, CoeffBitWidth=8, CoeffRound=1, TotalTaps=4, BitWidthIn=8, CoeffDistMem=1, WindowType=hamming, mult_latency=3, bram_latency=3, n_inputs=0, fwidth=1}
      mask prompts: nput "This is input number:"; PFBSize "Size of PFB: (2^? pnts)"; CoeffBitWidth "Bitwidth of Coefficients:"; CoeffRound "Round-off Coefficients:"; TotalTaps "Total Number of Taps:"; BitWidthIn "Input Bitwidth:"; CoeffDistMem "Implement Coeff Gen in Distributed Memory:"; WindowType "Windowing Function:"; mult_latency "Mult Latency"; bram_latency "BRAM Latency"; n_inputs "Number of Simultaneous Inputs: (2^?)"; fwidth "Bit Width (normal=1)"
      mask init:
      | first_tap_init(gcb,...
      |     'nput', nput,...
      |     'PFBSize', PFBSize,...
      |     'CoeffBitWidth', CoeffBitWidth,...
      |     'CoeffRound', CoeffRound,...
      |     'TotalTaps', TotalTaps,...
      |     'BitWidthIn', BitWidthIn,...
      |     'CoeffDistMem', CoeffDistMem,...
      |     'WindowType', WindowType,...
      |     'mult_latency', mult_latency,...
      |     'bram_latency', bram_latency,...
      |     'n_inputs', n_inputs,...
      |     'fwidth', fwidth);
      settings: AttributesFormatString=input=0, taps=4
      mask StyleString: edit,edit,edit,edit,edit,edit,edit,popup(bartlett|barthannwin|blackman|blackmanharris|bohamwin|chebwin|flattopwin|gausswin|hamming|hann|kaiser|nuttallwin|parzenwin|rectwin|tukeywin|triang),edit,edit,edit,edit
  pol1_in1_last_tap : Subsystem  AncestorBlock=casper_library/PFBs/last_tap  mask(last_tap){TotalTaps=4, BitWidthIn=8, BitWidthOut=18, CoeffBitWidth=8, add_latency=2, mult_latency=3, quantization=Truncate}
      mask prompts: TotalTaps "Total Number of Taps:"; BitWidthIn "Input Bitwidth:"; BitWidthOut "Output Bitwidth:"; CoeffBitWidth "Coeff Bitwidth:"; add_latency "Add Latency"; mult_latency "Mult Latency"; quantization "Quantization Behavior"
      mask init:
      | last_tap_init(gcb,...
      |     'TotalTaps', TotalTaps,...
      |     'BitWidthIn', BitWidthIn,...
      |     'BitWidthOut', BitWidthOut,...
      |     'CoeffBitWidth', CoeffBitWidth,...
      |     'add_latency', add_latency,...
      |     'mult_latency', mult_latency,...
      |     'quantization', quantization);
      settings: AttributesFormatString=taps=4
      mask StyleString: edit,edit,edit,edit,edit,edit,popup(Truncate|Round  (unbiased: +/- Inf)|Round  (unbiased: Even Values))
  pol1_in1_tap2 : casper_library/PFBs/tap
      link override delay/delay_bram/Constant2: equ=P=C
      link override sync_delay/Constant: equ=P=C
      link override sync_delay/Constant1: equ=P=C
      link override sync_delay/Constant2: equ=P=C
      link override sync_delay/Constant3: equ=P=C
  pol1_in1_tap3 : casper_library/PFBs/tap
      link override delay/delay_bram/Constant2: equ=P=C
      link override sync_delay/Constant: equ=P=C
      link override sync_delay/Constant1: equ=P=C
      link override sync_delay/Constant2: equ=P=C
      link override sync_delay/Constant3: equ=P=C
  pol2_in1_first_tap : Subsystem  AncestorBlock=casper_library/PFBs/first_tap  mask(first_tap){nput=0, PFBSize=11, CoeffBitWidth=8, CoeffRound=1, TotalTaps=4, BitWidthIn=8, CoeffDistMem=1, WindowType=hamming, mult_latency=3, bram_latency=3, n_inputs=0, fwidth=1}
      mask prompts: nput "This is input number:"; PFBSize "Size of PFB: (2^? pnts)"; CoeffBitWidth "Bitwidth of Coefficients:"; CoeffRound "Round-off Coefficients:"; TotalTaps "Total Number of Taps:"; BitWidthIn "Input Bitwidth:"; CoeffDistMem "Implement Coeff Gen in Distributed Memory:"; WindowType "Windowing Function:"; mult_latency "Mult Latency"; bram_latency "BRAM Latency"; n_inputs "Number of Simultaneous Inputs: (2^?)"; fwidth "Bit Width (normal=1)"
      mask init: same as ata_xaui_2048pt_w32pnk/pfb_fir1/pol1_in1_first_tap
      settings: AttributesFormatString=input=0, taps=4
      mask StyleString: edit,edit,edit,edit,edit,edit,edit,popup(bartlett|barthannwin|blackman|blackmanharris|bohamwin|chebwin|flattopwin|gausswin|hamming|hann|kaiser|nuttallwin|parzenwin|rectwin|tukeywin|triang),edit,edit,edit,edit
  pol2_in1_last_tap : Subsystem  AncestorBlock=casper_library/PFBs/last_tap  mask(last_tap){TotalTaps=4, BitWidthIn=8, BitWidthOut=18, CoeffBitWidth=8, add_latency=2, mult_latency=3, quantization=Truncate}
      mask prompts: TotalTaps "Total Number of Taps:"; BitWidthIn "Input Bitwidth:"; BitWidthOut "Output Bitwidth:"; CoeffBitWidth "Coeff Bitwidth:"; add_latency "Add Latency"; mult_latency "Mult Latency"; quantization "Quantization Behavior"
      mask init: same as ata_xaui_2048pt_w32pnk/pfb_fir1/pol1_in1_last_tap
      settings: AttributesFormatString=taps=4
      mask StyleString: edit,edit,edit,edit,edit,edit,popup(Truncate|Round  (unbiased: +/- Inf)|Round  (unbiased: Even Values))
  pol2_in1_tap2 : casper_library/PFBs/tap
      link override delay/delay_bram/Constant2: equ=P=C
      link override sync_delay/Constant: equ=P=C
      link override sync_delay/Constant1: equ=P=C
      link override sync_delay/Constant2: equ=P=C
      link override sync_delay/Constant3: equ=P=C
  pol2_in1_tap3 : casper_library/PFBs/tap
      link override delay/delay_bram/Constant2: equ=P=C
      link override sync_delay/Constant: equ=P=C
      link override sync_delay/Constant1: equ=P=C
      link override sync_delay/Constant2: equ=P=C
      link override sync_delay/Constant3: equ=P=C
  sync_out : Outport
  pol1_out1 : Outport  Port=2
  pol2_out1 : Outport  Port=3
  wires:
  pol1_in1/1 -> pol1_in1_first_tap/1(din)
  sync/1 -> pol1_in1_first_tap/2(sync), pol2_in1_first_tap/2(sync)
  pol1_in1_first_tap/1(dout) -> pol1_in1_tap2/1
  pol1_in1_first_tap/2(sync_out) -> pol1_in1_tap2/2
  pol1_in1_first_tap/3(coeff_out) -> pol1_in1_tap2/3
  pol1_in1_first_tap/4(taps_out) -> pol1_in1_tap2/4
  pol1_in1_tap2/1 -> pol1_in1_tap3/1
  pol1_in1_tap2/2 -> pol1_in1_tap3/2
  pol1_in1_tap2/3 -> pol1_in1_tap3/3
  pol1_in1_tap2/4 -> pol1_in1_tap3/4
  pol1_in1_tap3/1 -> pol1_in1_last_tap/1(din)
  pol1_in1_tap3/2 -> pol1_in1_last_tap/2(sync)
  pol1_in1_tap3/3 -> pol1_in1_last_tap/3(coeff)
  pol1_in1_tap3/4 -> pol1_in1_last_tap/4(taps)
  pol1_in1_last_tap/1(dout) -> pol1_out1/1
  pol1_in1_last_tap/2(sync_out) -> sync_out/1
  pol2_in1/1 -> pol2_in1_first_tap/1(din)
  pol2_in1_first_tap/1(dout) -> pol2_in1_tap2/1
  pol2_in1_first_tap/2(sync_out) -> pol2_in1_tap2/2
  pol2_in1_first_tap/3(coeff_out) -> pol2_in1_tap2/3
  pol2_in1_first_tap/4(taps_out) -> pol2_in1_tap2/4
  pol2_in1_tap2/1 -> pol2_in1_tap3/1
  pol2_in1_tap2/2 -> pol2_in1_tap3/2
  pol2_in1_tap2/3 -> pol2_in1_tap3/3
  pol2_in1_tap2/4 -> pol2_in1_tap3/4
  pol2_in1_tap3/1 -> pol2_in1_last_tap/1(din)
  pol2_in1_tap3/2 -> pol2_in1_last_tap/2(sync)
  pol2_in1_tap3/3 -> pol2_in1_last_tap/3(coeff)
  pol2_in1_tap3/4 -> pol2_in1_last_tap/4(taps)
  pol2_in1_last_tap/1(dout) -> pol2_out1/1

== system ata_xaui_2048pt_w32pnk/scope_s_output2 ==
  rst : Inport  Port=1  LatchInput=off
  en : Inport  Port=2  LatchInput=off
  data_in : Inport  Port=3  LatchInput=off
  Gateway Out : xbsIndex_r3/Gateway Out  output_type=Double  nbits=8  bin_pt=6  arith_type=Boolean  quantization=Truncate  overflow=Wrap  hdl_port=on  timing_constraint=None  locs_specified=off  LOCs={}  needs_fixed_name=off  show_param=off
      settings: xl_area=[0, 0, 0, 0, 0, 0, 0]
  Gateway Out1 : xbsIndex_r3/Gateway Out  output_type=Double  nbits=8  bin_pt=6  arith_type=Boolean  quantization=Truncate  overflow=Wrap  hdl_port=on  timing_constraint=None  locs_specified=off  LOCs={}  needs_fixed_name=off  show_param=off
      settings: xl_area=[0, 0, 0, 0, 0, 0, 0]
  Gateway Out2 : xbsIndex_r3/Gateway Out  output_type=Double  nbits=8  bin_pt=6  arith_type=Boolean  quantization=Truncate  overflow=Wrap  hdl_port=on  timing_constraint=None  locs_specified=off  LOCs={}  needs_fixed_name=off  show_param=off
      settings: xl_area=[0, 0, 0, 0, 0, 0, 0]
  Scope : Scope  NumInputPorts=3
      settings: YMin=-5~-5~-5  YMax=5~5~5
  bram : xps_library/Shared BRAM  Tag=xps:bram  arith_type="Signed  (2's comp)"  addr_width=11  data_width=32  data_bin_pt=23  init_vals=[1:2^11]  sample_rate=1
  freeze_cntr : casper_library/Misc/freeze_cntr  CounterBits=11
  wires:
  Gateway Out2/1 -> Scope/3
  Gateway Out1/1 -> Scope/2
  Gateway Out/1 -> Scope/1
  rst/1 -> freeze_cntr/2
  data_in/1 -> Gateway Out1/1, bram/2
  en/1 -> freeze_cntr/1
  freeze_cntr/2 -> Gateway Out2/1, bram/3
  freeze_cntr/1 -> Gateway Out/1, bram/1

== system ata_xaui_2048pt_w32pnk/scope_s_output3 ==
  rst : Inport  Port=1  LatchInput=off
  en : Inport  Port=2  LatchInput=off
  data_in : Inport  Port=3  LatchInput=off
  Gateway Out : xbsIndex_r3/Gateway Out  output_type=Double  nbits=8  bin_pt=6  arith_type=Boolean  quantization=Truncate  overflow=Wrap  hdl_port=on  timing_constraint=None  locs_specified=off  LOCs={}  needs_fixed_name=off  show_param=off
      settings: xl_area=[0, 0, 0, 0, 0, 0, 0]
  Gateway Out1 : xbsIndex_r3/Gateway Out  output_type=Double  nbits=8  bin_pt=6  arith_type=Boolean  quantization=Truncate  overflow=Wrap  hdl_port=on  timing_constraint=None  locs_specified=off  LOCs={}  needs_fixed_name=off  show_param=off
      settings: xl_area=[0, 0, 0, 0, 0, 0, 0]
  Gateway Out2 : xbsIndex_r3/Gateway Out  output_type=Double  nbits=8  bin_pt=6  arith_type=Boolean  quantization=Truncate  overflow=Wrap  hdl_port=on  timing_constraint=None  locs_specified=off  LOCs={}  needs_fixed_name=off  show_param=off
      settings: xl_area=[0, 0, 0, 0, 0, 0, 0]
  Scope : Scope  NumInputPorts=3
      settings: YMin=-5~-5~-5  YMax=5~5~5
  bram : xps_library/Shared BRAM  Tag=xps:bram  arith_type="Signed  (2's comp)"  addr_width=11  data_width=32  data_bin_pt=23  init_vals=[1:2^11]  sample_rate=1
  freeze_cntr : casper_library/Misc/freeze_cntr  CounterBits=11
  wires:
  freeze_cntr/1 -> bram/1, Gateway Out/1
  freeze_cntr/2 -> bram/3, Gateway Out2/1
  en/1 -> freeze_cntr/1
  data_in/1 -> bram/2, Gateway Out1/1
  rst/1 -> freeze_cntr/2
  Gateway Out/1 -> Scope/1
  Gateway Out1/1 -> Scope/2
  Gateway Out2/1 -> Scope/3
